simulink model "Car_7_Jan_takeoffandlanding_2012b"  (Simulink 8.0)
settings: Solver=ode5  StartTime=0.0  StopTime=inf  FixedStep=sample_time  RelTol=1e-3
InitFcn:
  | sample_time=0.005;%0.004;%0.0025;%0.02;
  | sample_time_Vicon = 0.005;
  | DeltaT = 0.02;
  | g = 9.81;
  | H0 = g%0.3165;
  | Kl = 1;
  | 
  | Q6_mass = 0.84;
  | 
  | Q6_Omega_r = 1.5; %for horizon ref
  | Q6_Zeta_r = 0.5; %for horizon ref
  | Q6_Omega_r_h = 2;%for vertical ref
  | Q6_Zeta_r_h = 2; %for vertical ref
  | 
  | 
  | Q6_Omega = 1.5; %for horizon control
  | Q6_Zeta = 0.5; %for horizon control
  | Q6_Omega_h= 2; %for vertical control
  | Q6_Zeta_h = 0.7; %for vertical control
  | 
  | 
  | Q6_acc_max = 5;%horizontal max acc
  | Q6_acc_max_h = 3;%horizontal max acc
  | 
  | omega_circle = 72*pi/180;
  | omega_h = 0.1;%Ascending speed
  | PI = pi;
  | Circle_R = 2.5;
  | MAX_Height = -2;
undefined symbols (not defined in the file or in its folder): DiscIntNeverNeededParam, fdesignblkfcn, gcbh
libraries: simulink x12, X330_Control x3, dspadpt3 x1
(part 2 of 2)

== matlab function UAV 1/Trajectory Logic/boundary ==
  data: PosDesiredx input double; newPosDesiredx output double; PosDesiredy input double; LPX input double; LPY input double; Posx input double; Posy input double; newPosDesiredy output double; desiredtopos output double
function [newPosDesiredx, newPosDesiredy,desiredtopos] = fcn(PosDesiredx,PosDesiredy, LPX,LPY,Posx,Posy)

UAVreal = [Posy, Posx,0];
UAVdesired = [PosDesiredy, PosDesiredx,0];
LA = [LPY, LPX,0];
r = 1.2;%%%%%landing_area circle radius
%%%%%%%%%%%%%%%%calculate point to line distance%%%%%%%%%%%
if(PosDesiredx == Posx && PosDesiredy == Posy)
    d = 1.3; %%%%%%%%%%%whatever value larger than 1.2, just for if this is not a line but a point
else
    a = UAVdesired - UAVreal;
    b = LA - UAVreal;
    d = norm(cross(a,b)) / norm(a);
end
%%%%%%%%%%%%%%%%%%%%%%%%%%%%%%%%%%%%%%%%%%%%%%%%%%%%%%%%%%
k = (PosDesiredx-Posx)/(PosDesiredy-Posy);
m = -k*PosDesiredy + PosDesiredx - LPX;
desiredtopos = sqrt((PosDesiredy-Posy)^2+(PosDesiredx-Posx)^2);
w = 0;
angleLAtoPos=atan2((Posx-LPX),(Posy-LPY));
if((Posx-LPX)^2+(Posy-LPY)^2<=r^2)%%%uav inside the circle already
    newPosDesiredx = LPX + r*cos(angleLAtoPos);
    newPosDesiredy = LPY + r*sin(angleLAtoPos);
else%%%%%%%uav outside the circle
if(d>=r)%%outside or tangent with circle
    n = 0;
    w = 0;
    zerochk = 0;
    wperpendicular = (w + 0.5 * pi)*zerochk;
    intersecty1 = Posy;
    intersecty2 = Posy;
    intersectx1 = Posx;
    intersectx2 = Posx;
    intersec1topos = sqrt((intersecty1-Posy)^2 + (intersectx1-Posx)^2);
    intersec2topos = sqrt((intersecty2-Posy)^2 + (intersectx2-Posx)^2);
    newPosDesiredy = PosDesiredy;
    newPosDesiredx = PosDesiredx;
else 
    n = sqrt(4*(LPY - k*m)^2 - 4*(k^2+1)*(LPY^2 + m^2 - r^2));
    intersecty1 = (2*(LPY - k*m)+n)/(2*(k^2+1));
    intersecty2 = (2*(LPY - k*m)-n)/(2*(k^2+1));
    intersectx1 = k*(intersecty1 - PosDesiredy)+PosDesiredx;
    intersectx2 = k*(intersecty2 - PosDesiredy)+PosDesiredx;
    intersec1topos = sqrt((intersecty1-Posy)^2 + (intersectx1-Posx)^2);
    intersec2topos = sqrt((intersecty2-Posy)^2 + (intersectx2-Posx)^2);
    if(intersec1topos<intersec2topos)
        w = atan2((LPX-intersectx1),(LPY-intersecty1));
    else
        w = atan2((LPX-intersectx2),(LPY-intersecty2));
    end
        if(desiredtopos<=intersec1topos && desiredtopos<=intersec2topos)
            newPosDesiredx = PosDesiredx;
            newPosDesiredy = PosDesiredy;
            zerochk = 0;
            wperpendicular = (w + 0.5 * pi)*zerochk;
        elseif(desiredtopos<=intersec1topos && desiredtopos>intersec2topos)
            newPosDesiredx = intersectx2;
            newPosDesiredy = intersecty2;
            zerochk = 0;
            wperpendicular = (w + 0.5 * pi)*zerochk;
        elseif(desiredtopos>intersec1topos && desiredtopos<=intersec2topos)  
            newPosDesiredx = intersectx1;
            newPosDesiredy = intersecty1;
            zerochk = 0;
            wperpendicular = (w + 0.5 * pi)*zerochk;
        else
            zerochk = 1;
            wperpendicular = (w + 0.5 * pi)*zerochk;
            if(intersec1topos<intersec2topos)
            newPosDesiredx = 0.5*cos(wperpendicular) + intersectx1;
            newPosDesiredy = 0.5*sin(wperpendicular) + intersecty1;
            else
            newPosDesiredx = 0.5*cos(wperpendicular) + intersectx2;
            newPosDesiredy = 0.5*sin(wperpendicular) + intersecty2;  
            end
            
        end
    
end 
end

== matlab function UAV 1/Trajectory Logic/masscontrol ==
  data: match_flag output double; posx input double; posy input double; posz input double; Cpx input double; mass output double; Cpy input double; Cpz input double; mass_flag input double
function [match_flag,mass] = fcn(posx,posy,posz,Cpx,Cpy,Cpz,mass_flag)
%#codegen
if(abs(Cpx-posx)+abs(Cpy-posy)<0.3)
    match_flag = 1;
else
    match_flag = 0;
end
if(mass_flag == 1)%match_flag==1 && Cpz<=-0.07 &&
    mass = 1.2;
else
    mass = 0.92;
end

== stateflow chart UAV 1/Trajectory Logic/stateflowforwholesequence ==
  state Landing
    state CutThrottle
      du:HoverThrottle = (0.0 - HoverThrottle)*2*DeltaT + HoverThrottle ;
    state Decsending
      du:PosDesired[2] = (landing_area[2] - PosDesired[2])*1*DeltaT + PosDesired[2] ;
    (default) -> Landing.Decsending
    Landing.Decsending -> Landing.CutThrottle : [Pos[2] > landing_area[2]-0.05]
  state Airborne1
    state TakeOff
      du:HoverThrottle = (H0 - HoverThrottle)*2*DeltaT + HoverThrottle ;
    state capturing_sequence_success
      state movetoLAfinish2
        du: PosDesired[2] = -1.3; PosDesired[0] = landing_area[0];PosDesired[1] = landing_area[1];
      state caputuring_test
        en: PosDesired = Pos; PosDesired[2] = -1.3;
      state prepare_move_LA2
        du: smooth_flag = 1;PosDesired[2] = -1.3; PosDesired[0] = 0;PosDesired[1] = 0;
      state movetoLA2
        du: PosDesired[2] = -1.3; PosDesired[0] = landing_area[0];PosDesired[1] = 0;
      (default) -> caputuring_test
      caputuring_test -> prepare_move_LA2 : after(5,sec)
      prepare_move_LA2 -> movetoLA2 : after(5,sec)
      movetoLA2 -> movetoLAfinish2 : after(5,sec)
    state Hover
      en: PosDesired[2] = -1.3;
    state Hover1
      en: PosDesired[2] = -1.3;
    state movetoorigin
      en: PosDesired[0] = landing_area[0]; PosDesired[1] = 0;
    state movetoorigin1
      en: PosDesired[0] =0; PosDesired[1] = 0;
    state capturing
      state normal_capturing3
        en: PosDesired[0] = car[0] ; PosDesired[1] = car[1]; PosDesired[2] = -0.5;
      state normal_capturing4
        en: PosDesired[0] = carest[0] + 0.2*(car[0] - Pos[0])/abs(car[0] - Pos[0]); PosDesired[1] = carest[1] + 0.2*(car[1] - Pos[1])/(abs(car[1] - Pos[1])); PosDesired[2] = -0.5;
      (default) -> normal_capturing3
      normal_capturing4 -> normal_capturing3 : after(1,sec)
      normal_capturing3 -> normal_capturing4 : after(1,sec)
    (default) -> TakeOff : {smooth_flag =1;mass_flag = 0;PosDesired = Pos;PosDesired[2] = -1; }
    TakeOff -> Hover : after(5,sec)
    Hover -> movetoorigin : after(8,sec)
    movetoorigin -> movetoorigin1 : after(5,sec)
    capturing_sequence_success -> capturing : [RC[5] < 0]
        | {PosDesired = Pos;smooth_flag = 0;mass_flag = 0;}
    movetoorigin1 -> Hover1 : after(5,sec)
    capturing -> capturing_sequence_success : [RC[5] > 0]
        | {smooth_flag = 1;mass_flag = 1;}
    Hover1 -> capturing : after(5,sec)
        | {smooth_flag = 0;}
  state prepare_move_LA
    du: PosDesired[2] = -1.3; PosDesired[0] = 0;PosDesired[1] = 0;
  state movetoLA
    du: PosDesired[2] = -1.3; PosDesired[0] = landing_area[0];PosDesired[1] = 0;
  state movetoLAfinish
    du: PosDesired[2] = -1.3; PosDesired[0] = landing_area[0];PosDesired[1] = landing_area[1];
  state Decsending
    du:PosDesired[2] = (-0.8 - PosDesired[2])*1*DeltaT + PosDesired[2] ;
  state CutThrottle
    du:HoverThrottle = (0.01 - HoverThrottle)*2*DeltaT + HoverThrottle ;
  state tracking_mode
    du: PosDesired[2] = -0.6; PosDesired[0] = car[0];PosDesired[1] = car[1];
  Landing -> Airborne1 : [RC[6] > 0.5]
  Airborne1 -> Landing : [RC[6] < -0.5]
  prepare_move_LA -> movetoLA : after(5,sec)
  movetoLA -> movetoLAfinish : after(5,sec)
  movetoLAfinish -> Decsending : [(abs(Pos[0]-PosDesired[0])+abs(Pos[1]-PosDesired[1]))<0.02]
  (default) -> Landing : {HoverThrottle=0.01;}
  Decsending -> CutThrottle : [Pos[2] > -0.8]
  data: PosDesired output double size=4; HoverThrottle output double size=1; RC input double size=8; Pos input double size=4; DeltaT parameter double size=1; H0 parameter double size=1; Kl parameter double size=1; VelCmd local double size=2 =0; line_count local int8 size=1 =0; triangle_count local int8 size=1 =0; T_line local double size=1; omega_circle parameter double size=1; PI parameter double size=1; omega_h parameter double; Circle_R parameter double size=1; MAX_Height parameter double size=1; landing_area input double size=6; car input double size=6; carest input double size=2; match_flag input double; smooth_flag output boolean =0; matchx local double; matchy local double; mass_flag output boolean
